simulink model "Exercitiul4"  (R2016a)
settings: Solver=VariableStepAuto  StartTime=0.0  StopTime=480  RelTol=1e-3
undefined symbols (not defined in the file): m, n
settings Model: Creator=Cristina  LastModifiedBy=Cristina

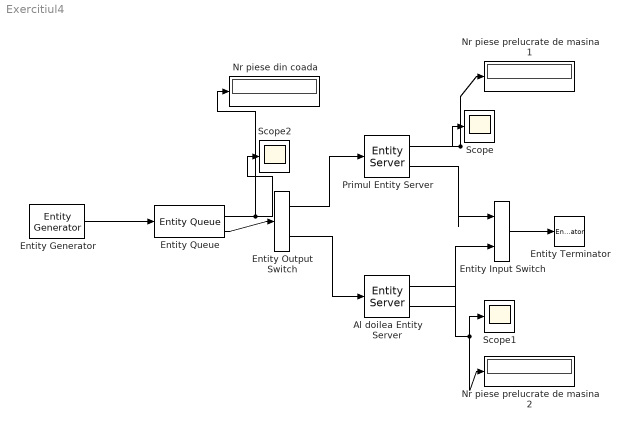
== system Exercitiul4 ==
  Al doilea Entity Server : EntityServer  InputPortMessageModes=m  OutputPortMessageModes=n,m  Capacity=1  ServiceTimeValue=1.1  NumberEntitiesDeparted=on
      settings: OutputPortMap=o0,o9
  Entity Input Switch : EntityInputSwitch  InputPortMessageModes=m,m  OutputPortMessageModes=m
  Entity Output Switch : EntityOutputSwitch  InputPortMessageModes=m  OutputPortMessageModes=m,m  SwitchingCriterion=From attribute  SwitchAttributeName=prt
  Entity Generator : EntityGenerator  OutputPortMessageModes=m  Period=0.5  AttributeName=prt  AttributeInitialValue=3  EntityType=Structured  EntityTypeName=Entity
  Entity Queue : EntityQueue  InputPortMessageModes=m  OutputPortMessageModes=n,m  EntryAction=|  NumberEntitiesInBlock=on
      | if rand < 0.5
      |     entity.prt = 2;
      | else
      |     entity.prt = 1;
      | end
      settings: OutputPortMap=o1,o5
  Entity Terminator : EntityTerminator  InputPortMessageModes=m
  Nr piese din coada : Display
  Nr piese prelucrate de masina 1 : Display
  Nr piese prelucrate de masina 2 : Display
  Primul Entity Server : EntityServer  InputPortMessageModes=m  OutputPortMessageModes=n,m  Capacity=1  ServiceTimeValue=0.9  NumberEntitiesDeparted=on
      settings: OutputPortMap=o0,o9
  Scope : Scope
  Scope1 : Scope
  Scope2 : Scope
  wires:
  Entity Generator/1 -> Entity Queue/1
  Entity Queue/2 -> Entity Output Switch/1
  Entity Output Switch/1 -> Primul Entity Server/1
  Entity Output Switch/2 -> Al doilea Entity Server/1
  Primul Entity Server/2 -> Entity Input Switch/1
  Al doilea Entity Server/2 -> Entity Input Switch/2
  Entity Input Switch/1 -> Entity Terminator/1
  Primul Entity Server/1 -> Nr piese prelucrate de masina 1/1, Scope/1
  Al doilea Entity Server/1 -> Scope1/1, Nr piese prelucrate de masina 2/1
  Entity Queue/1 -> Nr piese din coada/1, Scope2/1
